simulink model "DRFO"  (R2014a)
settings: Solver=ode23tb  StartTime=0.0  StopTime=1  RelTol=1e-6
libraries: powerlib x4, powerlib_meascontrol x4, simulink x3
settings Model: Creator=ninad gaikawad  LastModifiedBy=ninad gaikawad
settings SolverCC: ZeroCrossControl=DisableAll  SolverResetMethod=Robust

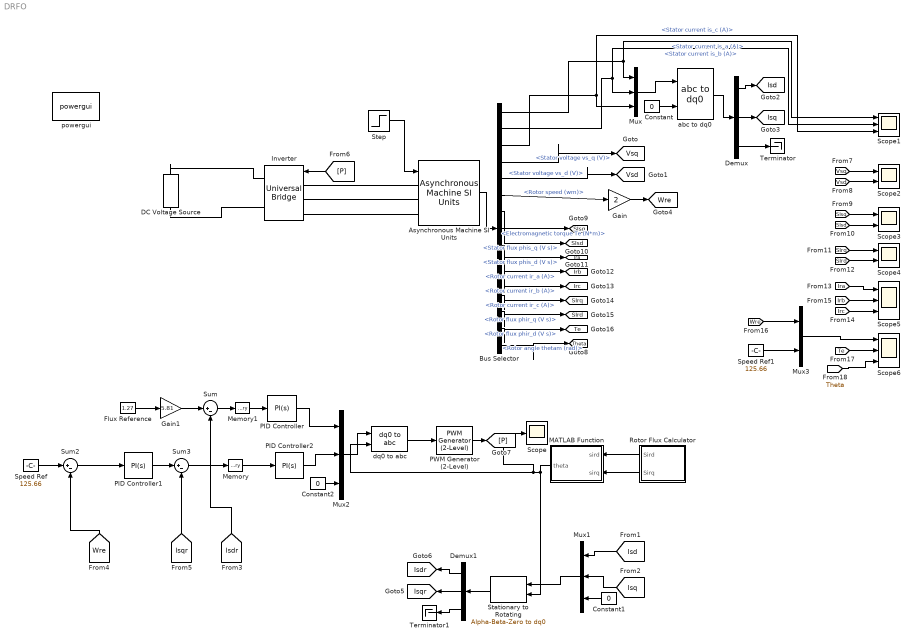
== system DRFO ==
  Asynchronous Machine SI Units : powerlib/Machines/Asynchronous Machine SI Units  PresetModel="15:  5.4 HP (4KW)   400 V  50Hz 1430 RPM"  MechanicalLoad=Torque Tm  ShowDetailedParameters=on  RotorType=Squirrel-cage  ReferenceFrame=Rotor  Units=SI  MeasurementBus=off  NominalParameters=[4000 400 50]  Stator=[1.405 0.005839]  Rotor=[1.395 0.005839]  Cage1=[ 0.022 0.226/377]  Cage2=[ 0.022 0.226/377]  Lm=0.1722  Mechanical=[0.0131 0.002985 2]  PolePairs=2  InitialConditions=[1 0 0 0 0 0 0 0]  SimulateSaturation=off  Saturation=[14.03593122, 27.81365428, 53.79336849, 72.68890987, 97.98006896, 148.6815601, 215.7428561, 302.9841135, 420.4778367 ; 230, 322, 414, 460, 506, 552, 598, 644, 690]  LoadFlowParameters=1492000  TsPowergui=0  TsBlock=-1  IterativeModel=Trapezoidal non iterative  Pmec=0
  Bus Selector : BusSelector  OutputSignals=Stator measurements.Stator current is_a (A),Stator measurements.Stator current is_b (A),Stator measurements.Stator current is_c (A),Stator measurements.Stator voltage vs_q (V),Stator measurements.Stator voltage vs_d (V),Mechanical.Rotor speed (wm),Mechanical.Electromagnetic torque Te (N*m),Stator measurements.Stator flux phis_q (V s),Stator measurements.Stator flux phis_d (V s),Rotor measurements.Rotor current ir_a (A),Rotor measurements.Rotor current ir_b (A),Rotor measurements.Rotor current ir_c (A),Rotor measurements.Rotor flux phir_q (V s),Rotor measurements.Rotor flux phir_d (V s),Mechanical.Rotor angle thetam (rad)
  Constant : Constant  Value=0
  Constant1 : Constant  Value=0
  Constant2 : Constant  Value=0
  DC Voltage Source : powerlib/Electrical Sources/DC Voltage Source  Amplitude=624  Measurements=None
  Demux : Demux  Outputs=3
  Demux1 : Demux  Outputs=3
  Flux Reference : Constant  Value=1.27
  Gain : Gain  Gain=2
  Gain1 : Gain  Gain=5.81
  Inverter : powerlib/Power Electronics/Universal Bridge  Arms=3  SnubberResistance=1e5  SnubberCapacitance=inf  Device=IGBT / Diodes  Ron=1e-3  Lon=0  ForwardVoltages="[  0  0  ]"  ForwardVoltage=0  GTOparameters=[ 10e-6 , 20e-6 ]  IGBTparameters=[ 1e-6 , 2e-6 ]  Measurements=None  Measurements_2=None  converterType=Rectifier
  MATLAB Function : MATLAB Function  TreatAsAtomicUnit=on
  Memory : Memory  X0=1  InheritSampleTime=on  LinearizeAsDelay=on
  Memory1 : Memory  X0=0.2  InheritSampleTime=on  LinearizeAsDelay=on
  Mux : Mux  Inputs=3
  Mux1 : Mux  Inputs=3
  Mux2 : Mux  Inputs=3
  Mux3 : Mux  Inputs=2
  PID Controller : simulink/Continuous/PID Controller  Controller=PI  TimeDomain=Continuous-time  SampleTime=1  IntegratorMethod=Forward Euler  FilterMethod=Forward Euler  Form=Parallel  P=0.45  I=1  D=0  N=100  InitialConditionSource=internal  InitialConditionForIntegrator=0  InitialConditionForFilter=0  ExternalReset=none  LimitOutput=on  UpperSaturationLimit=1  LowerSaturationLimit=0  LinearizeAsGain=on  AntiWindupMode=clamping  Kb=1  TrackingMode=off  Kt=1  PParamMin=[]  PParamMax=[]  IParamMin=[]  IParamMax=[]  DParamMin=[]  DParamMax=[]  NParamMin=[]  NParamMax=[]  KbParamMin=[]  KbParamMax=[]  KtParamMin=[]  KtParamMax=[]  POutMin=[]  POutMax=[]  IOutMin=[]  IOutMax=[]  DOutMin=[]  DOutMax=[]  NOutMin=[]  NOutMax=[]  KbOutMin=[]  KbOutMax=[]  KtOutMin=[]  KtOutMax=[]  IntegratorOutMin=[]  IntegratorOutMax=[]  FilterOutMin=[]  FilterOutMax=[]  SumOutMin=[]  SumOutMax=[]  SumI1OutMin=[]  SumI1OutMax=[]  SumI2OutMin=[]  SumI2OutMax=[]  SumI3OutMin=[]  SumI3OutMax=[]  SumDOutMin=[]  SumDOutMax=[]  SaturationOutMin=[]  SaturationOutMax=[]  IntegratorContinuousStateAttributes=''  IntegratorStateMustResolveToSignalObject=off  IntegratorRTWStateStorageClass=Auto  FilterContinuousStateAttributes=''  FilterStateMustResolveToSignalObject=off  FilterRTWStateStorageClass=Auto
  PID Controller1 : simulink/Continuous/PID Controller  Controller=PI  TimeDomain=Continuous-time  SampleTime=1  IntegratorMethod=Forward Euler  FilterMethod=Forward Euler  Form=Parallel  P=1  I=1  D=0  N=100  InitialConditionSource=internal  InitialConditionForIntegrator=0  InitialConditionForFilter=0  ExternalReset=none  LimitOutput=off  UpperSaturationLimit=1  LowerSaturationLimit=-1  LinearizeAsGain=on  AntiWindupMode=clamping  Kb=1  TrackingMode=off  Kt=1  PParamMin=[]  PParamMax=[]  IParamMin=[]  IParamMax=[]  DParamMin=[]  DParamMax=[]  NParamMin=[]  NParamMax=[]  KbParamMin=[]  KbParamMax=[]  KtParamMin=[]  KtParamMax=[]  POutMin=[]  POutMax=[]  IOutMin=[]  IOutMax=[]  DOutMin=[]  DOutMax=[]  NOutMin=[]  NOutMax=[]  KbOutMin=[]  KbOutMax=[]  KtOutMin=[]  KtOutMax=[]  IntegratorOutMin=[]  IntegratorOutMax=[]  FilterOutMin=[]  FilterOutMax=[]  SumOutMin=[]  SumOutMax=[]  SumI1OutMin=[]  SumI1OutMax=[]  SumI2OutMin=[]  SumI2OutMax=[]  SumI3OutMin=[]  SumI3OutMax=[]  SumDOutMin=[]  SumDOutMax=[]  SaturationOutMin=[]  SaturationOutMax=[]  IntegratorContinuousStateAttributes=''  IntegratorStateMustResolveToSignalObject=off  IntegratorRTWStateStorageClass=Auto  FilterContinuousStateAttributes=''  FilterStateMustResolveToSignalObject=off  FilterRTWStateStorageClass=Auto
  PID Controller2 : simulink/Continuous/PID Controller  Controller=PI  TimeDomain=Continuous-time  SampleTime=1  IntegratorMethod=Forward Euler  FilterMethod=Forward Euler  Form=Parallel  P=1  I=1  D=0  N=100  InitialConditionSource=internal  InitialConditionForIntegrator=0  InitialConditionForFilter=0  ExternalReset=none  LimitOutput=on  UpperSaturationLimit=1  LowerSaturationLimit=0  LinearizeAsGain=on  AntiWindupMode=clamping  Kb=1  TrackingMode=off  Kt=1  PParamMin=[]  PParamMax=[]  IParamMin=[]  IParamMax=[]  DParamMin=[]  DParamMax=[]  NParamMin=[]  NParamMax=[]  KbParamMin=[]  KbParamMax=[]  KtParamMin=[]  KtParamMax=[]  POutMin=[]  POutMax=[]  IOutMin=[]  IOutMax=[]  DOutMin=[]  DOutMax=[]  NOutMin=[]  NOutMax=[]  KbOutMin=[]  KbOutMax=[]  KtOutMin=[]  KtOutMax=[]  IntegratorOutMin=[]  IntegratorOutMax=[]  FilterOutMin=[]  FilterOutMax=[]  SumOutMin=[]  SumOutMax=[]  SumI1OutMin=[]  SumI1OutMax=[]  SumI2OutMin=[]  SumI2OutMax=[]  SumI3OutMin=[]  SumI3OutMax=[]  SumDOutMin=[]  SumDOutMax=[]  SaturationOutMin=[]  SaturationOutMax=[]  IntegratorContinuousStateAttributes=''  IntegratorStateMustResolveToSignalObject=off  IntegratorRTWStateStorageClass=Auto  FilterContinuousStateAttributes=''  FilterStateMustResolveToSignalObject=off  FilterRTWStateStorageClass=Auto
  PWM Generator (2-Level) : powerlib_meascontrol/Pulse & Signal Generators/PWM Generator (2-Level)  ModulatorType=Three-phase bridge (6 pulses)  ModulatorMode=Unsynchronized  nF=27  Fc=1000  ModulatingSignals=off  m=0.8  Freq=60  Phase=0  Ts=0
  Rotor Flux Calculator : Subsystem
  Scope : Scope
      settings: YMin=-3.5  YMax=3.5
  Scope1 : Scope  NumInputPorts=3
      settings: YMin=-5~-5~-5  YMax=5~5~5
  Scope2 : Scope  NumInputPorts=2
      settings: YMin=-5~-5  YMax=5~5  SaveName=ScopeData2
  Scope3 : Scope  NumInputPorts=2
      settings: YMin=-5~-5  YMax=5~5  SaveName=ScopeData3
  Scope4 : Scope  NumInputPorts=2
      settings: TimeRange=0.25  YMin=-10~0.17  YMax=15~0.27  SaveName=ScopeData4
  Scope5 : Scope  NumInputPorts=3
      settings: YMin=-5~-5~-5  YMax=5~5~5  SaveName=ScopeData5
  Scope6 : Scope  NumInputPorts=3
      settings: YMin=-6500~-0.003~-3168  YMax=500~0.003~-3154  SaveName=ScopeData6
  Speed Ref : Constant  Value=125.66
  Speed Ref1 : Constant  Value=125.66
  Stationary to Rotating : powerlib_meascontrol/Transformations/Alpha-Beta-Zero to dq0  Alignment=Aligned with phase A axis
  Step : Step  Time=0.5  After=26.71  SampleTime=0
  Sum : Sum  Inputs=|+-
  Sum2 : Sum  Inputs=|+-
  Sum3 : Sum  Inputs=|+-
  Terminator : Terminator
  Terminator1 : Terminator
  abc to dq0 : powerlib_meascontrol/Transformations/abc to dq0  Alignment=Aligned with phase A axis
  dq0 to abc : powerlib_meascontrol/Transformations/dq0 to abc  Alignment=Aligned with phase A axis
  powergui : powerlib/powergui  Priority=1  SimulationMode=Continuous  SolverType=Tustin  SampleTime=50e-6  frequency=60  SPID=off  DisableSnubberDevices=off  DisableRonSwitches=off  DisableVfSwitches=off  SwTol=0  Interpol=off  DisplayEquations=off  Ts=0  methode=off  frequencyindice=50  Pbase=100e6  ErrMax=1e-4  Iterations=50  UnitsV=kV  UnitsW=MW  FunctionMessages=off  echomessages=off  HookPort=off  EnableUseOfTLC=off  x0status=blocks  RestoreLinks=warning  ResistiveCurrentMeasurement=off  Frange=[0:2:500]  Ylog=off  Xlog=on  ShowGrid=off  save=off  variable=ZData  structure=0  ZoomFFT=off  StartTime=0.0  cycles=1  DisplayStyle=1  fundamental=60  FreqAxis=off  MaxFrequency=1000  frequencyindicesteady=1  RmsSteady=1  display=off
  tag scope: Ira=global, Irb=global, Irc=global, Isd=global, Isdr=global, Isq=global, Isqr=global, SIrd=global, SIrq=global, SIsd=global, SIsq=global, Te=global, Theta=global, Vsd=global, Vsq=global, Wre=global
  wires:
  Asynchronous Machine SI Units/1 -> Bus Selector/1
  Bus Selector/1 -> Scope1/1, Mux/1  "<Stator current is_a (A)>"
  Bus Selector/2 -> Scope1/2, Mux/2  "<Stator current is_b (A)>"
  Bus Selector/3 -> Scope1/3, Mux/3  "<Stator current is_c (A)>"
  Mux/1 -> abc to dq0/1
  abc to dq0/1 -> Demux/1
  Demux/3 -> Terminator/1
  Bus Selector/6 -> Gain/1  "<Rotor speed (wm)>"
  Demux/2 -> [Isq]
  Demux/1 -> [Isd]
  Bus Selector/4 -> [Vsq]  "<Stator voltage vs_q (V)>"
  Bus Selector/5 -> [Vsd]  "<Stator voltage vs_d (V)>"
  Gain/1 -> [Wre]
  Constant/1 -> abc to dq0/2
  [Isd] -> Mux1/1
  [Isq] -> Mux1/2
  Constant1/1 -> Mux1/3
  Mux1/1 -> Stationary to Rotating/1
  MATLAB Function/1(theta) -> Scope/1, dq0 to abc/2, Stationary to Rotating/2
  Stationary to Rotating/1 -> Demux1/1
  Demux1/3 -> Terminator1/1
  Demux1/2 -> [Isqr]
  Demux1/1 -> [Isdr]
  PID Controller1/1 -> Sum3/1
  Speed Ref/1 -> Sum2/1
  PID Controller/1 -> Mux2/1
  PID Controller2/1 -> Mux2/2
  Constant2/1 -> Mux2/3
  Mux2/1 -> dq0 to abc/1
  dq0 to abc/1 -> PWM Generator (2-Level)/1
  PWM Generator (2-Level)/1 -> [P]
  [P] -> Inverter/1
  Gain1/1 -> Sum/1
  Flux Reference/1 -> Gain1/1
  Step/1 -> Asynchronous Machine SI Units/1
  Sum2/1 -> PID Controller1/1
  Sum3/1 -> Memory/1
  Memory/1 -> PID Controller2/1
  Sum/1 -> Memory1/1
  Memory1/1 -> PID Controller/1
  [Wre] -> Sum2/2
  [Isqr] -> Sum3/2
  [Isdr] -> Sum/2
  Bus Selector/7 -> [SIsq]  "<Electromagnetic torque Te (N*m)>"
  Bus Selector/8 -> [SIsd]  "<Stator flux phis_q (V s)>"
  Bus Selector/9 -> [Ira]  "<Stator flux phis_d (V s)>"
  Bus Selector/10 -> [Irb]  "<Rotor current ir_a (A)>"
  Bus Selector/11 -> [Irc]  "<Rotor current ir_b (A)>"
  Bus Selector/12 -> [SIrq]  "<Rotor current ir_c (A)>"
  Bus Selector/13 -> [SIrd]  "<Rotor flux phir_q (V s)>"
  Bus Selector/14 -> [Te]  "<Rotor flux phir_d (V s)>"
  Bus Selector/15 -> [Theta]  "<Rotor angle thetam (rad)>"
  [Te] -> Scope6/2
  [Irc] -> Scope5/3
  [Irb] -> Scope5/2
  [Ira] -> Scope5/1
  [SIrd] -> Scope4/2
  [SIrq] -> Scope4/1
  [SIsd] -> Scope3/2
  [SIsq] -> Scope3/1
  [Vsd] -> Scope2/2
  [Vsq] -> Scope2/1
  Speed Ref1/1 -> Mux3/2
  [Theta] -> Scope6/3
  [Wre] -> Mux3/1
  Mux3/1 -> Scope6/1
  Rotor Flux Calculator/1(Sird) -> MATLAB Function/1(sird)
  Rotor Flux Calculator/2(Sirq) -> MATLAB Function/2(sirq)
  connections:
  DC Voltage Source/RConn1 -- Inverter/RConn1
  DC Voltage Source/LConn1 -- Inverter/RConn2
  Inverter/LConn1 -- Asynchronous Machine SI Units/LConn1
  Inverter/LConn2 -- Asynchronous Machine SI Units/LConn2
  Inverter/LConn3 -- Asynchronous Machine SI Units/LConn3

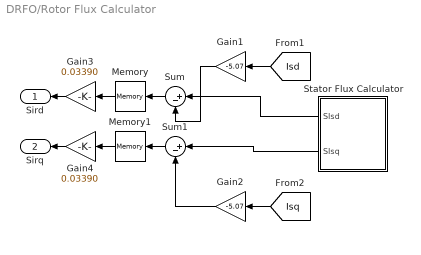
== system DRFO/Rotor Flux Calculator ==
  Gain1 : Gain  Gain=-5.07
  Gain2 : Gain  Gain=-5.07
  Gain3 : Gain  Gain=0.03390
  Gain4 : Gain  Gain=0.03390
  Memory : Memory  X0=1
  Memory1 : Memory  X0=1
  Stator Flux Calculator : Subsystem
  Sum : Sum  Inputs=|+-
  Sum1 : Sum  Inputs=|+-
  Sird : Outport
  Sirq : Outport  Port=2
  wires:
  Gain1/1 -> Sum/2
  [Isq] -> Gain2/1
  Gain2/1 -> Sum1/2
  Stator Flux Calculator/1(SIsd) -> Sum/1
  Stator Flux Calculator/2(SIsq) -> Sum1/1
  Sum1/1 -> Memory1/1
  [Isd] -> Gain1/1
  Sum/1 -> Memory/1
  Gain3/1 -> Sird/1
  Gain4/1 -> Sirq/1
  Memory/1 -> Gain3/1
  Memory1/1 -> Gain4/1

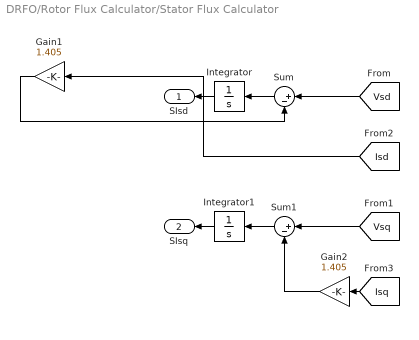
== system DRFO/Rotor Flux Calculator/Stator Flux Calculator ==
  Gain1 : Gain  Gain=1.405
  Gain2 : Gain  Gain=1.405
  Integrator : Integrator
  Integrator1 : Integrator
  Sum : Sum  Inputs=|+-
  Sum1 : Sum  Inputs=|+-
  SIsd : Outport
  SIsq : Outport  Port=2
  wires:
  Gain2/1 -> Sum1/2
  [Isq] -> Gain2/1
  Sum/1 -> Integrator/1
  Gain1/1 -> Sum/2
  Sum1/1 -> Integrator1/1
  [Vsd] -> Sum/1
  [Vsq] -> Sum1/1
  [Isd] -> Gain1/1
  Integrator/1 -> SIsd/1
  Integrator1/1 -> SIsq/1

== matlab function DRFO/MATLAB Function ==
  settings: updateMethod=CONTINUOUS
  data: sird input; theta output; sirq input
function theta = func(sird,sirq)
theta=atan2(sirq,sird);
